simulink model "Copy_of_ADRCSi_TST"  (R2021b)
settings: Solver=ode4  StartTime=0.0  StopTime=14.895  FixedStep=0.003  RelTol=1e-3
InitFcn:
  | T_set=2;
  | b0=1/(13.1);
  | T_sam=0.003;
  | s_cl=-6/T_set;
  | s_eso=1.5*s_cl;
  | z_eso=exp(s_eso*T_sam);
  | Kd=-2*s_cl;
  | Kp=(s_cl)^2;
  | l1=-3*s_eso;
  | l2=3*(s_eso)^2;
  | l3=-(s_eso)^3;
  | 
  | 
  | %Thong so Notch filter
  | w0=4.337;
  | D=0.0001;
  | T_set1=3;
  | b01=1/(0.87);
  | T_sam1=0.003;
  | s_cl1=-6/T_set1;
  | s_eso1=20*s_cl1;
  | z_eso1=exp(s_eso1*T_sam1);
  | Kd1=-2*s_cl1;
  | Kp1=(s_cl1)^2;
  | l11=-3*s_eso1;
  | l21=3*(s_eso1)^2;
  | l31=-(s_eso1)^3;
StopFcn:
  | close all;
  | 
  | B = [100, 100, 600 300];
  | figure('Position', B);
  | figure(1)
  | hold on;
  | plot(out.tout,out.F1,'linewidth',1.2);
  | %plot(out.tout,out.F11,'linewidth',1.2);
  | %plot(out.tout,out.F12,'linewidth',1.2);
  | %plot(out.tout,out.F13,'linewidth',1.2);
  | legend('ADRC', 'ADRC+ZV','ADRC+ZVD','ADRC+ETM4');
  | xlabel('Thời gian (s)');
  | ylabel('F1 (N)');
  | grid on
  | 
  | % do thi vi tri
  | figure('Position', B);
  | figure(2)
  | plot(out.tout,out.X1,'linewidth',1.2);
  | plot(out.tout,out.X11,'linewidth',1.2);
  | plot(out.tout,out.X12,'linewidth',1.2);
  | plot(out.tout,out.X13,'linewidth',1.2);
  | hold on
  | grid on
  | xlabel('Thời gian (s)');
  | ylabel('x1 (m)');
  | legend('ADRC');
  | 
  | % do thi dao dong diem giua
  | figure('Position', B);
  | figure(3)
  | hold on
  | grid on
  | plot(out.tout,out.W_MID,'linewidth',1.2);
  | plot(out.tout,out.W_MID1,'--r','linewidth',1.2);
  | plot(out.tout,out.W_MID2,'-.k','linewidth',1.2);
  | plot(out.tout,out.W_MID3,'-m','linewidth',1.2);
  | xlabel('Thời gian (s)');
  | ylabel('ω(L/2, t)(m)');
  | legend('ADRC', 'ADRC+ZV','ADRC+ZVD','ADRC+ETM4');
  | 
  | % do thi dao dong diem cuoi
  | figure('Position', B);
  | figure(4)
  | hold on
  | grid on
  | plot(out.tout,out.WL,'linewidth',0.7);
  | plot(out.tout,out.WL1,'linewidth',0.7);
  | plot(out.tout,out.WL2,'linewidth',0.7);
  | plot(out.tout,out.WL3,'linewidth',0.7);
  | xlabel('Thời gian (s)');
  | ylabel('ω(L,t) (m)');
  | legend('Middle point','End point');
  | axis([0 15 -0.04 0.04])
  | legend('ADRC', 'ADRC+ZV','ADRC+ZVD','ADRC+ETM4');
  | 
  | %do thi pho tan so
  | figure('Position', B);
  | tmax = 15;
  | r = 5000;
  | dt = tmax/(r);
  | Fs=1/dt;
  | time=0:dt:(r-2)*dt-dt;
  | l1=r;
  | grid on
  | hold on
  | 
  | fft_w=fft(out.W_MID,l1)*(2/l1);
  | abs_w=abs(fft_w);
  | freq=0:(1/time(end)):Fs/2-(1/time(end));
  | plot(freq,abs_w(1:length(freq)),LineWidth=1.2);
  | 
  | fft_w=fft(out.WL,l1)*(2/l1);
  | abs_w=abs(fft_w);
  | freq=0:(1/time(end)):Fs/2-(1/time(end));
  | plot(freq,abs_w(1:length(freq)),LineWidth=1.2);
  | xlabel('Tần số (Hz)');
  | ylabel('Biên độ (m)')
  | legend('Middle point','End point');
  | A = [0 10 0 0.02 ];
  | axis(A);
settings Model: Creator=Admin  LastModifiedBy=ADMIN

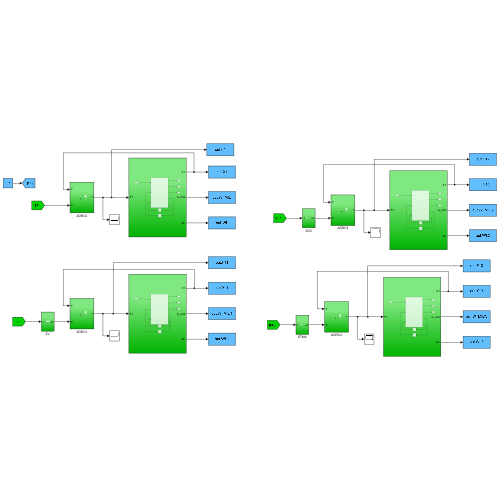
[thumbnail: Simulink's stored preview of the top-level diagram]
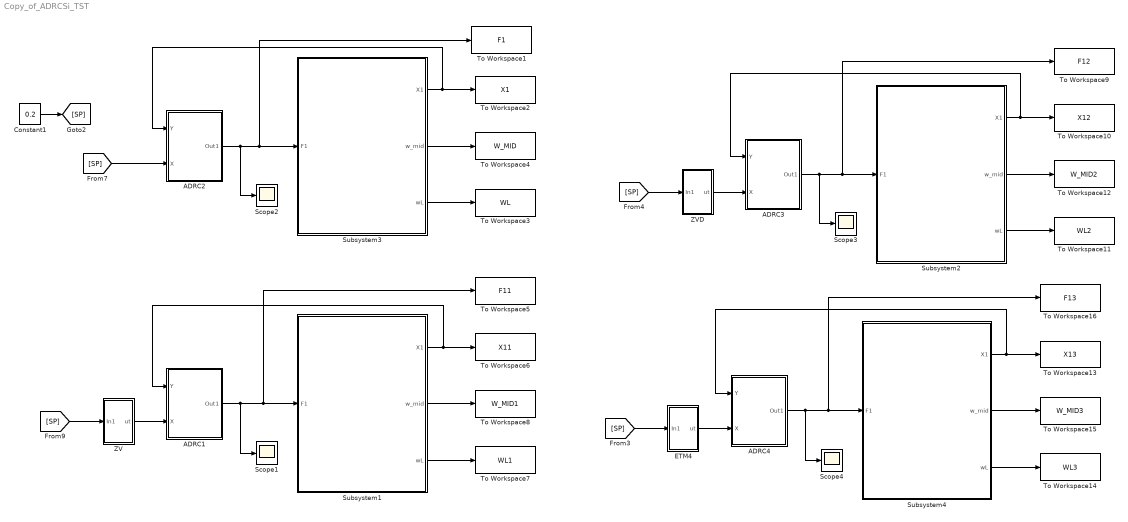
== system Copy_of_ADRCSi_TST ==
  ADRC1 : Subsystem
  ADRC2 : Subsystem
  ADRC3 : Subsystem
  ADRC4 : Subsystem
  Constant1 : Constant  Value=0.2
  ETM4 : Subsystem
  Scope{1..4} (4 alike) : Scope
  Subsystem1 : Subsystem
  Subsystem2 : Subsystem
  Subsystem3 : Subsystem
  Subsystem4 : Subsystem
  To Workspace1 : ToWorkspace  VariableName=F1  SampleTime=-1
      settings: Save2DSignal=2-D array (concatenate along first dimension)
  To Workspace10 : ToWorkspace  VariableName=X12  SampleTime=-1
      settings: Save2DSignal=2-D array (concatenate along first dimension)
  To Workspace11 : ToWorkspace  VariableName=WL2  SampleTime=-1
      settings: Save2DSignal=2-D array (concatenate along first dimension)
  To Workspace12 : ToWorkspace  VariableName=W_MID2  SampleTime=-1
      settings: Save2DSignal=2-D array (concatenate along first dimension)
  To Workspace13 : ToWorkspace  VariableName=X13  SampleTime=-1
      settings: Save2DSignal=2-D array (concatenate along first dimension)
  To Workspace14 : ToWorkspace  VariableName=WL3  SampleTime=-1
      settings: Save2DSignal=2-D array (concatenate along first dimension)
  To Workspace15 : ToWorkspace  VariableName=W_MID3  SampleTime=-1
      settings: Save2DSignal=2-D array (concatenate along first dimension)
  To Workspace16 : ToWorkspace  VariableName=F13  SampleTime=-1
      settings: Save2DSignal=2-D array (concatenate along first dimension)
  To Workspace2 : ToWorkspace  VariableName=X1  SampleTime=-1
      settings: Save2DSignal=2-D array (concatenate along first dimension)
  To Workspace3 : ToWorkspace  VariableName=WL  SampleTime=-1
      settings: Save2DSignal=2-D array (concatenate along first dimension)
  To Workspace4 : ToWorkspace  VariableName=W_MID  SampleTime=-1
      settings: Save2DSignal=2-D array (concatenate along first dimension)
  To Workspace5 : ToWorkspace  VariableName=F11  SampleTime=-1
      settings: Save2DSignal=2-D array (concatenate along first dimension)
  To Workspace6 : ToWorkspace  VariableName=X11  SampleTime=-1
      settings: Save2DSignal=2-D array (concatenate along first dimension)
  To Workspace7 : ToWorkspace  VariableName=WL1  SampleTime=-1
      settings: Save2DSignal=2-D array (concatenate along first dimension)
  To Workspace8 : ToWorkspace  VariableName=W_MID1  SampleTime=-1
      settings: Save2DSignal=2-D array (concatenate along first dimension)
  To Workspace9 : ToWorkspace  VariableName=F12  SampleTime=-1
      settings: Save2DSignal=2-D array (concatenate along first dimension)
  ZV : Subsystem
  ZVD : Subsystem
  wires:
  Subsystem3/1(X1) -> ADRC2/1(Y), To Workspace2/1
  [SP] -> ADRC2/2(X)
  ADRC2/1(Out1) -> To Workspace1/1, Subsystem3/1(F1), Scope2/1
  Constant1/1 -> [SP]
  Subsystem3/2(w_mid) -> To Workspace4/1
  Subsystem1/2(w_mid) -> To Workspace8/1
  ADRC1/1(Out1) -> To Workspace5/1, Subsystem1/1(F1), Scope1/1
  Subsystem1/3(wL) -> To Workspace7/1
  Subsystem1/1(X1) -> ADRC1/1(Y), To Workspace6/1
  [SP] -> ZV/1(In1)
  ZV/1(ut) -> ADRC1/2(X)
  ZVD/1(ut) -> ADRC3/2(X)
  [SP] -> ZVD/1(In1)
  Subsystem2/1(X1) -> ADRC3/1(Y), To Workspace10/1
  ADRC3/1(Out1) -> To Workspace9/1, Subsystem2/1(F1), Scope3/1
  Subsystem2/2(w_mid) -> To Workspace12/1
  Subsystem2/3(wL) -> To Workspace11/1
  [SP] -> ETM4/1(In1)
  ETM4/1(ut) -> ADRC4/2(X)
  ADRC4/1(Out1) -> To Workspace16/1, Subsystem4/1(F1), Scope4/1
  Subsystem4/1(X1) -> ADRC4/1(Y), To Workspace13/1
  Subsystem4/2(w_mid) -> To Workspace15/1
  Subsystem4/3(wL) -> To Workspace14/1
  Subsystem3/3(wL) -> To Workspace3/1

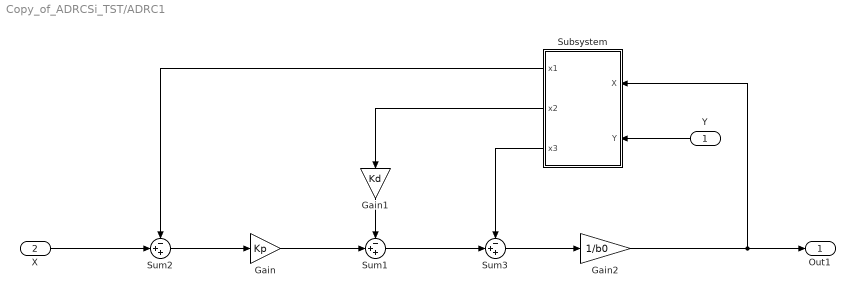
== system Copy_of_ADRCSi_TST/ADRC1 ==
  Y : Inport
  X : Inport  Port=2
  Gain : Gain  Gain=Kp
  Gain1 : Gain  Gain=Kd
  Gain2 : Gain  Gain=1/b0
  Subsystem : Subsystem
  Sum1 : Sum  Inputs=-++
  Sum2 : Sum  Inputs=-++
  Sum3 : Sum  Inputs=-++
  Out1 : Outport
  wires:
  Sum1/1 -> Sum3/2
  Subsystem/1(x1) -> Sum2/1
  Sum3/1 -> Gain2/1
  Gain/1 -> Sum1/2
  Subsystem/3(x3) -> Sum3/1
  Gain1/1 -> Sum1/1
  Gain2/1 -> Out1/1, Subsystem/1(X)
  Subsystem/2(x2) -> Gain1/1
  Sum2/1 -> Gain/1
  Y/1 -> Subsystem/2(Y)
  X/1 -> Sum2/2

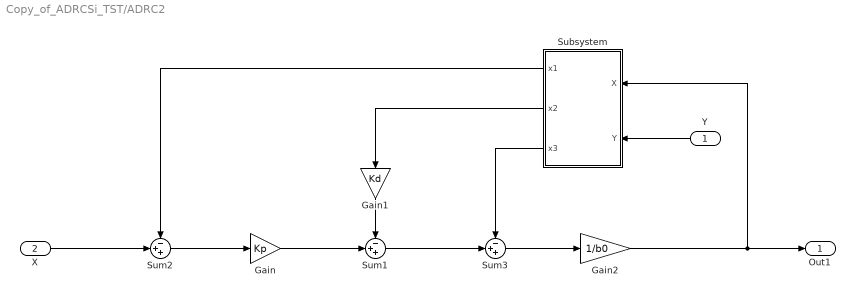
== system Copy_of_ADRCSi_TST/ADRC2 ==
  Y : Inport
  X : Inport  Port=2
  Gain : Gain  Gain=Kp
  Gain1 : Gain  Gain=Kd
  Gain2 : Gain  Gain=1/b0
  Subsystem : Subsystem
  Sum1 : Sum  Inputs=-++
  Sum2 : Sum  Inputs=-++
  Sum3 : Sum  Inputs=-++
  Out1 : Outport
  wires:
  Sum1/1 -> Sum3/2
  Subsystem/1(x1) -> Sum2/1
  Sum3/1 -> Gain2/1
  Gain/1 -> Sum1/2
  Subsystem/3(x3) -> Sum3/1
  Gain1/1 -> Sum1/1
  Gain2/1 -> Out1/1, Subsystem/1(X)
  Subsystem/2(x2) -> Gain1/1
  Sum2/1 -> Gain/1
  Y/1 -> Subsystem/2(Y)
  X/1 -> Sum2/2

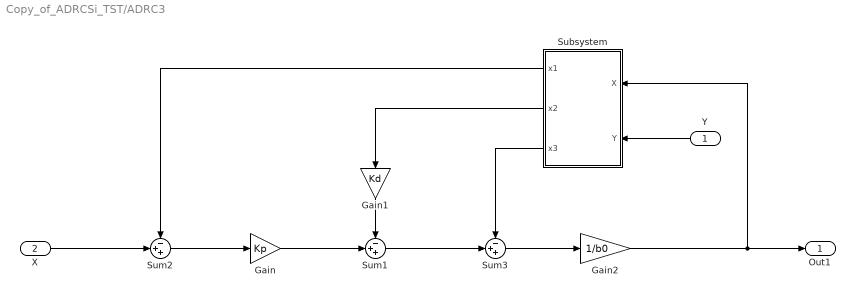
== system Copy_of_ADRCSi_TST/ADRC3 ==
  Y : Inport
  X : Inport  Port=2
  Gain : Gain  Gain=Kp
  Gain1 : Gain  Gain=Kd
  Gain2 : Gain  Gain=1/b0
  Subsystem : Subsystem
  Sum1 : Sum  Inputs=-++
  Sum2 : Sum  Inputs=-++
  Sum3 : Sum  Inputs=-++
  Out1 : Outport
  wires:
  Sum1/1 -> Sum3/2
  Subsystem/1(x1) -> Sum2/1
  Sum3/1 -> Gain2/1
  Gain/1 -> Sum1/2
  Subsystem/3(x3) -> Sum3/1
  Gain1/1 -> Sum1/1
  Gain2/1 -> Out1/1, Subsystem/1(X)
  Subsystem/2(x2) -> Gain1/1
  Sum2/1 -> Gain/1
  Y/1 -> Subsystem/2(Y)
  X/1 -> Sum2/2

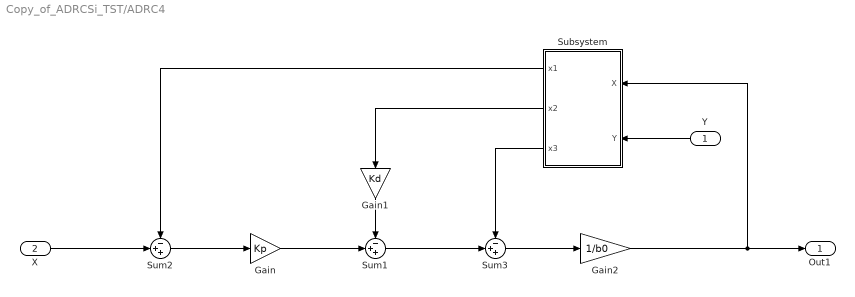
== system Copy_of_ADRCSi_TST/ADRC4 ==
  Y : Inport
  X : Inport  Port=2
  Gain : Gain  Gain=Kp
  Gain1 : Gain  Gain=Kd
  Gain2 : Gain  Gain=1/b0
  Subsystem : Subsystem
  Sum1 : Sum  Inputs=-++
  Sum2 : Sum  Inputs=-++
  Sum3 : Sum  Inputs=-++
  Out1 : Outport
  wires:
  Sum1/1 -> Sum3/2
  Subsystem/1(x1) -> Sum2/1
  Sum3/1 -> Gain2/1
  Gain/1 -> Sum1/2
  Subsystem/3(x3) -> Sum3/1
  Gain1/1 -> Sum1/1
  Gain2/1 -> Out1/1, Subsystem/1(X)
  Subsystem/2(x2) -> Gain1/1
  Sum2/1 -> Gain/1
  Y/1 -> Subsystem/2(Y)
  X/1 -> Sum2/2

== system Copy_of_ADRCSi_TST/ETM4 ==
  In1 : Inport
  ETM : Subsystem
  ut : Outport
  wires:
  In1/1 -> ETM/1(In1)
  ETM/1(ut) -> ut/1

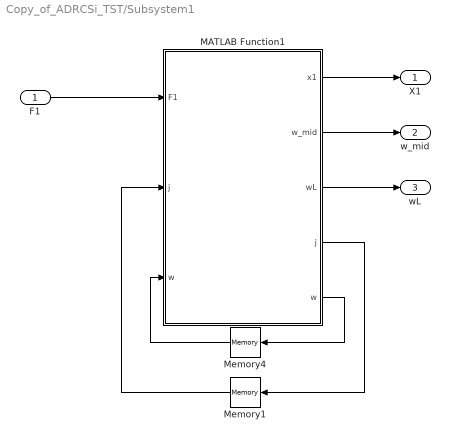
== system Copy_of_ADRCSi_TST/Subsystem1 ==
  F1 : Inport
  MATLAB Function1 : MATLAB Function  TreatAsAtomicUnit=on
  Memory1 : Memory
  Memory4 : Memory  InitialCondition=zeros(15,10000)
  X1 : Outport
  w_mid : Outport  Port=2
  wL : Outport  Port=3
  wires:
  Memory4/1 -> MATLAB Function1/3("w ")
  Memory1/1 -> MATLAB Function1/2("j ")
  MATLAB Function1/4(j) -> Memory1/1
  MATLAB Function1/5(w) -> Memory4/1
  MATLAB Function1/3(wL) -> wL/1
  F1/1 -> MATLAB Function1/1(F1)
  MATLAB Function1/1(x1) -> X1/1
  MATLAB Function1/2(w_mid) -> w_mid/1

== system Copy_of_ADRCSi_TST/Subsystem2 ==
  F1 : Inport
  MATLAB Function1 : MATLAB Function  TreatAsAtomicUnit=on
  Memory1 : Memory
  Memory4 : Memory  InitialCondition=zeros(15,10000)
  X1 : Outport
  w_mid : Outport  Port=2
  wL : Outport  Port=3
  wires:
  Memory4/1 -> MATLAB Function1/3("w ")
  Memory1/1 -> MATLAB Function1/2("j ")
  MATLAB Function1/4(j) -> Memory1/1
  MATLAB Function1/5(w) -> Memory4/1
  MATLAB Function1/3(wL) -> wL/1
  F1/1 -> MATLAB Function1/1(F1)
  MATLAB Function1/1(x1) -> X1/1
  MATLAB Function1/2(w_mid) -> w_mid/1

== system Copy_of_ADRCSi_TST/Subsystem3 ==
  F1 : Inport
  MATLAB Function1 : MATLAB Function  TreatAsAtomicUnit=on
  Memory1 : Memory
  Memory4 : Memory  InitialCondition=zeros(15,10000)
  X1 : Outport
  w_mid : Outport  Port=2
  wL : Outport  Port=3
  wires:
  Memory4/1 -> MATLAB Function1/3("w ")
  Memory1/1 -> MATLAB Function1/2("j ")
  MATLAB Function1/4(j) -> Memory1/1
  MATLAB Function1/5(w) -> Memory4/1
  MATLAB Function1/3(wL) -> wL/1
  F1/1 -> MATLAB Function1/1(F1)
  MATLAB Function1/1(x1) -> X1/1
  MATLAB Function1/2(w_mid) -> w_mid/1

== system Copy_of_ADRCSi_TST/Subsystem4 ==
  F1 : Inport
  MATLAB Function1 : MATLAB Function  TreatAsAtomicUnit=on
  Memory1 : Memory
  Memory4 : Memory  InitialCondition=zeros(15,10000)
  X1 : Outport
  w_mid : Outport  Port=2
  wL : Outport  Port=3
  wires:
  Memory4/1 -> MATLAB Function1/3("w ")
  Memory1/1 -> MATLAB Function1/2("j ")
  MATLAB Function1/4(j) -> Memory1/1
  MATLAB Function1/5(w) -> Memory4/1
  MATLAB Function1/3(wL) -> wL/1
  F1/1 -> MATLAB Function1/1(F1)
  MATLAB Function1/1(x1) -> X1/1
  MATLAB Function1/2(w_mid) -> w_mid/1

== system Copy_of_ADRCSi_TST/ZV ==
  In1 : Inport
  IS4 : Subsystem
  ut : Outport
  wires:
  In1/1 -> IS4/1(In1)
  IS4/1(ut) -> ut/1

== system Copy_of_ADRCSi_TST/ZVD ==
  In1 : Inport
  IS4_7 : Subsystem
  ut : Outport
  wires:
  In1/1 -> IS4_7/1(In1)
  IS4_7/1(ut) -> ut/1

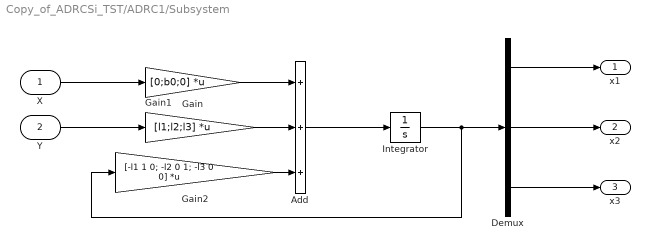
== system Copy_of_ADRCSi_TST/ADRC1/Subsystem ==
  X : Inport
  Y : Inport  Port=2
  Add : Sum  Inputs=+++
  Demux : Demux  Outputs=3
  Gain : Gain  Gain=[0;b0;0]  Multiplication=Matrix(K*u)
  Gain1 : Gain  Gain=[l1;l2;l3]  Multiplication=Matrix(K*u)
  Gain2 : Gain  Gain=[-l1 1 0; -l2 0 1; -l3 0 0]  Multiplication=Matrix(K*u)
  Integrator : Integrator
  x1 : Outport
  x2 : Outport  Port=2
  x3 : Outport  Port=3
  wires:
  Gain1/1 -> Add/2
  Demux/3 -> x3/1
  Demux/1 -> x1/1
  Gain2/1 -> Add/3
  Demux/2 -> x2/1
  Gain/1 -> Add/1
  Add/1 -> Integrator/1
  Integrator/1 -> Gain2/1, Demux/1
  Y/1 -> Gain1/1
  X/1 -> Gain/1

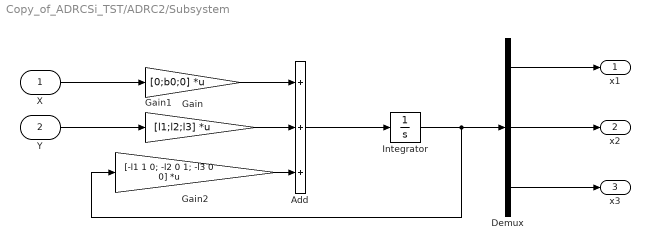
== system Copy_of_ADRCSi_TST/ADRC2/Subsystem ==
  X : Inport
  Y : Inport  Port=2
  Add : Sum  Inputs=+++
  Demux : Demux  Outputs=3
  Gain : Gain  Gain=[0;b0;0]  Multiplication=Matrix(K*u)
  Gain1 : Gain  Gain=[l1;l2;l3]  Multiplication=Matrix(K*u)
  Gain2 : Gain  Gain=[-l1 1 0; -l2 0 1; -l3 0 0]  Multiplication=Matrix(K*u)
  Integrator : Integrator
  x1 : Outport
  x2 : Outport  Port=2
  x3 : Outport  Port=3
  wires:
  Gain1/1 -> Add/2
  Demux/3 -> x3/1
  Demux/1 -> x1/1
  Gain2/1 -> Add/3
  Demux/2 -> x2/1
  Gain/1 -> Add/1
  Add/1 -> Integrator/1
  Integrator/1 -> Gain2/1, Demux/1
  Y/1 -> Gain1/1
  X/1 -> Gain/1

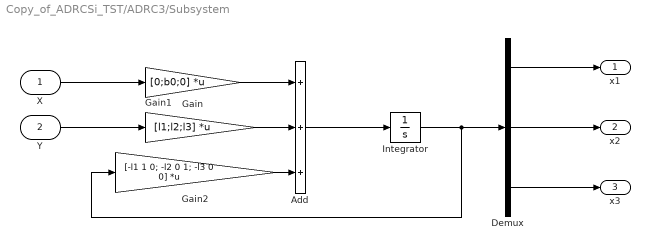
== system Copy_of_ADRCSi_TST/ADRC3/Subsystem ==
  X : Inport
  Y : Inport  Port=2
  Add : Sum  Inputs=+++
  Demux : Demux  Outputs=3
  Gain : Gain  Gain=[0;b0;0]  Multiplication=Matrix(K*u)
  Gain1 : Gain  Gain=[l1;l2;l3]  Multiplication=Matrix(K*u)
  Gain2 : Gain  Gain=[-l1 1 0; -l2 0 1; -l3 0 0]  Multiplication=Matrix(K*u)
  Integrator : Integrator
  x1 : Outport
  x2 : Outport  Port=2
  x3 : Outport  Port=3
  wires:
  Gain1/1 -> Add/2
  Demux/3 -> x3/1
  Demux/1 -> x1/1
  Gain2/1 -> Add/3
  Demux/2 -> x2/1
  Gain/1 -> Add/1
  Add/1 -> Integrator/1
  Integrator/1 -> Gain2/1, Demux/1
  Y/1 -> Gain1/1
  X/1 -> Gain/1

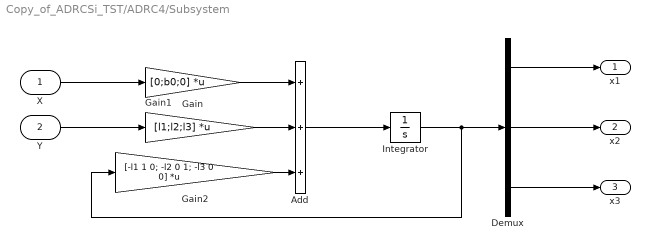
== system Copy_of_ADRCSi_TST/ADRC4/Subsystem ==
  X : Inport
  Y : Inport  Port=2
  Add : Sum  Inputs=+++
  Demux : Demux  Outputs=3
  Gain : Gain  Gain=[0;b0;0]  Multiplication=Matrix(K*u)
  Gain1 : Gain  Gain=[l1;l2;l3]  Multiplication=Matrix(K*u)
  Gain2 : Gain  Gain=[-l1 1 0; -l2 0 1; -l3 0 0]  Multiplication=Matrix(K*u)
  Integrator : Integrator
  x1 : Outport
  x2 : Outport  Port=2
  x3 : Outport  Port=3
  wires:
  Gain1/1 -> Add/2
  Demux/3 -> x3/1
  Demux/1 -> x1/1
  Gain2/1 -> Add/3
  Demux/2 -> x2/1
  Gain/1 -> Add/1
  Add/1 -> Integrator/1
  Integrator/1 -> Gain2/1, Demux/1
  Y/1 -> Gain1/1
  X/1 -> Gain/1

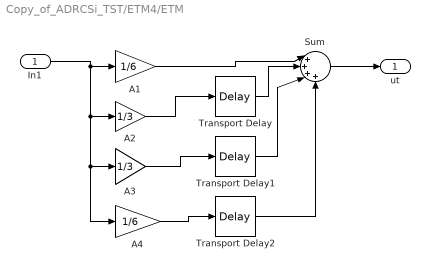
== system Copy_of_ADRCSi_TST/ETM4/ETM ==
  In1 : Inport
  A1 : Gain  Gain=1/6
  A2 : Gain  Gain=1/3
  A3 : Gain  Gain=1/3
  A4 : Gain  Gain=1/6
  Sum : Sum  Inputs=|++++
  Transport Delay : TransportDelay  DelayTime=1/1.73437/3
  Transport Delay1 : TransportDelay  DelayTime=1/1.73437*2/3
  Transport Delay2 : TransportDelay  DelayTime=1/1.73437
  ut : Outport
  wires:
  Sum/1 -> ut/1
  Transport Delay/1 -> Sum/2
  A2/1 -> Transport Delay/1
  A1/1 -> Sum/1
  A3/1 -> Transport Delay1/1
  Transport Delay1/1 -> Sum/3
  In1/1 -> A4/1, A3/1, A2/1, A1/1
  A4/1 -> Transport Delay2/1
  Transport Delay2/1 -> Sum/4

== system Copy_of_ADRCSi_TST/ZV/IS4 ==
  In1 : Inport
  A1 : Gain  Gain=0.5
  A2 : Gain  Gain=0.5
  Sum : Sum  Inputs=|++
  Transport Delay : TransportDelay  DelayTime=1/(2*1.73437)
  ut : Outport
  wires:
  Sum/1 -> ut/1
  In1/1 -> A2/1, A1/1
  Transport Delay/1 -> Sum/2
  A2/1 -> Transport Delay/1
  A1/1 -> Sum/1

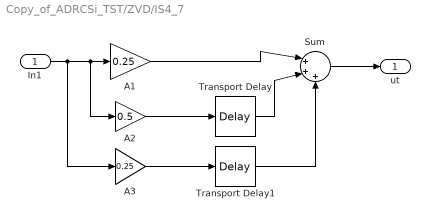
== system Copy_of_ADRCSi_TST/ZVD/IS4_7 ==
  In1 : Inport
  A1 : Gain  Gain=0.25
  A2 : Gain  Gain=0.5
  A3 : Gain  Gain=0.25
  Sum : Sum  Inputs=|+++
  Transport Delay : TransportDelay  DelayTime=1/(2*1.73437)
  Transport Delay1 : TransportDelay  DelayTime=1/(1.73437)
  ut : Outport
  wires:
  Sum/1 -> ut/1
  Transport Delay/1 -> Sum/2
  A2/1 -> Transport Delay/1
  A1/1 -> Sum/1
  A3/1 -> Transport Delay1/1
  In1/1 -> A3/1, A1/1, A2/1
  Transport Delay1/1 -> Sum/3

== matlab function Copy_of_ADRCSi_TST/Subsystem1/MATLAB Function1 ==
  data: F1 input; x1 output; w_mid output; wL output; j input; j output; w input; w output
function [x1,w_mid,wL,j,w]= fcn(F1,j,w)
%nhap so lieu cua dam`
k=1;
pA=2.4882;EI=0.236;g=9.81;
%pA=2.4882;EI=0.1635;g=9.81;
% pA=2.4882;EI=1.05;g=9.81;
L=0.6;
mw=13.1;
mk=0.2;
% cac buoc sai phan
tmax=15;
r=5000;
dt=tmax/r;
n=9;% so diem chia => chia thanh thanh 5 diem 
ds=L/(n-1); 
S1=(EI*(dt^2))/(mw*(ds^3));
S2=(-EI*(dt^2))/((ds^4)*pA);
S3=(EI*(dt^2))/(mk*2*ds^3);
j=j+1;
% mo phong diem x1
S1=(EI*dt^2)/(mw*ds^3);
wsss01=(w(3,j+1)-2*w(2,j+1)+w(1,j+1))/(2*ds^3);
w(1,j+2)=(F1-EI*wsss01)*(dt^2/mw)+2*w(1,j+1)-w(1,j);
w(2,j+2)=w(1,j+2);
for i=3:n-2
S2=(-EI*dt^2)/(ds^4*pA);
wssss=w(i+2,j+1)-4*w(i+1,j+1)+6*w(i,j+1)-4*w(i-1,j+1)+w(i-2,j+1);
w(i,j+2)=S2*wssss+2*w(i,j+1)-w(i,j);
end
wsssl=(-2*w(n,j+1)+3*w(n-1,j+1)-w(n-2,j+1));
w(n,j+2)=2*w(n,j+1)-w(n,j)+S3*wsssl;
w(n-1,j+2)=(w(n,j+2)+w(n-2,j+2))/2;
x1=w(1,j);
wL=w(n,j)-w(1,j);
w_mid=w(5,j)-w(1,j);
end

== matlab function Copy_of_ADRCSi_TST/Subsystem2/MATLAB Function1 ==
  data: F1 input; x1 output; w_mid output; wL output; j input; j output; w input; w output
function [x1,w_mid,wL,j,w]= fcn(F1,j,w)
%nhap so lieu cua dam`
k=1;
pA=2.4882;EI=0.236;g=9.81;
%pA=2.4882;EI=0.1635;g=9.81;
% pA=2.4882;EI=1.05;g=9.81;
L=0.6;
mw=13.1;
mk=0.2;
% cac buoc sai phan
tmax=15;
r=5000;
dt=tmax/r;
n=9;% so diem chia => chia thanh thanh 5 diem 
ds=L/(n-1); 
S1=(EI*(dt^2))/(mw*(ds^3));
S2=(-EI*(dt^2))/((ds^4)*pA);
S3=(EI*(dt^2))/(mk*2*ds^3);
j=j+1;
% mo phong diem x1
S1=(EI*dt^2)/(mw*ds^3);
wsss01=(w(3,j+1)-2*w(2,j+1)+w(1,j+1))/(2*ds^3);
w(1,j+2)=(F1-EI*wsss01)*(dt^2/mw)+2*w(1,j+1)-w(1,j);
w(2,j+2)=w(1,j+2);
for i=3:n-2
S2=(-EI*dt^2)/(ds^4*pA);
wssss=w(i+2,j+1)-4*w(i+1,j+1)+6*w(i,j+1)-4*w(i-1,j+1)+w(i-2,j+1);
w(i,j+2)=S2*wssss+2*w(i,j+1)-w(i,j);
end
wsssl=(-2*w(n,j+1)+3*w(n-1,j+1)-w(n-2,j+1));
w(n,j+2)=2*w(n,j+1)-w(n,j)+S3*wsssl;
w(n-1,j+2)=(w(n,j+2)+w(n-2,j+2))/2;
x1=w(1,j);
wL=w(n,j)-w(1,j);
w_mid=w(5,j)-w(1,j);
end

== matlab function Copy_of_ADRCSi_TST/Subsystem3/MATLAB Function1 ==
  data: F1 input; x1 output; w_mid output; wL output; j input; j output; w input; w output
function [x1,w_mid,wL,j,w]= fcn(F1,j,w)
%nhap so lieu cua dam`
k=1;
pA=2.4882;EI=0.236;g=9.81;
%pA=2.4882;EI=0.1635;g=9.81;
% pA=2.4882;EI=1.05;g=9.81;
L=0.6;
mw=13.1;
mk=0.2;
% cac buoc sai phan
tmax=15;
r=5000;
dt=tmax/r;
n=9;% so diem chia => chia thanh thanh 5 diem 
ds=L/(n-1); 
S1=(EI*(dt^2))/(mw*(ds^3));
S2=(-EI*(dt^2))/((ds^4)*pA);
S3=(EI*(dt^2))/(mk*2*ds^3);
j=j+1;
% mo phong diem x1
S1=(EI*dt^2)/(mw*ds^3);
wsss01=(w(3,j+1)-2*w(2,j+1)+w(1,j+1))/(2*ds^3);
w(1,j+2)=(F1-EI*wsss01)*(dt^2/mw)+2*w(1,j+1)-w(1,j);
w(2,j+2)=w(1,j+2);
for i=3:n-2
S2=(-EI*dt^2)/(ds^4*pA);
wssss=w(i+2,j+1)-4*w(i+1,j+1)+6*w(i,j+1)-4*w(i-1,j+1)+w(i-2,j+1);
w(i,j+2)=S2*wssss+2*w(i,j+1)-w(i,j);
end
wsssl=(-2*w(n,j+1)+3*w(n-1,j+1)-w(n-2,j+1));
w(n,j+2)=2*w(n,j+1)-w(n,j)+S3*wsssl;
w(n-1,j+2)=(w(n,j+2)+w(n-2,j+2))/2;
x1=w(1,j);
wL=w(n,j)-w(1,j);
w_mid=w(5,j)-w(1,j);
end

== matlab function Copy_of_ADRCSi_TST/Subsystem4/MATLAB Function1 ==
  data: F1 input; x1 output; w_mid output; wL output; j input; j output; w input; w output
function [x1,w_mid,wL,j,w]= fcn(F1,j,w)
%nhap so lieu cua dam`
k=1;
pA=2.4882;EI=0.236;g=9.81;
%pA=2.4882;EI=0.1635;g=9.81;
% pA=2.4882;EI=1.05;g=9.81;
L=0.6;
mw=13.1;
mk=0.2;
% cac buoc sai phan
tmax=15;
r=5000;
dt=tmax/r;
n=9;% so diem chia => chia thanh thanh 5 diem 
ds=L/(n-1); 
S1=(EI*(dt^2))/(mw*(ds^3));
S2=(-EI*(dt^2))/((ds^4)*pA);
S3=(EI*(dt^2))/(mk*2*ds^3);
j=j+1;
% mo phong diem x1
S1=(EI*dt^2)/(mw*ds^3);
wsss01=(w(3,j+1)-2*w(2,j+1)+w(1,j+1))/(2*ds^3);
w(1,j+2)=(F1-EI*wsss01)*(dt^2/mw)+2*w(1,j+1)-w(1,j);
w(2,j+2)=w(1,j+2);
for i=3:n-2
S2=(-EI*dt^2)/(ds^4*pA);
wssss=w(i+2,j+1)-4*w(i+1,j+1)+6*w(i,j+1)-4*w(i-1,j+1)+w(i-2,j+1);
w(i,j+2)=S2*wssss+2*w(i,j+1)-w(i,j);
end
wsssl=(-2*w(n,j+1)+3*w(n-1,j+1)-w(n-2,j+1));
w(n,j+2)=2*w(n,j+1)-w(n,j)+S3*wsssl;
w(n-1,j+2)=(w(n,j+2)+w(n-2,j+2))/2;
x1=w(1,j);
wL=w(n,j)-w(1,j);
w_mid=w(5,j)-w(1,j);
end
